simulink model "pendulum3"  (R2020b)
settings: Solver=VariableStepAuto  StartTime=0.0  StopTime=20  RelTol=1e-3
settings Model: Creator=Admin  LastModifiedBy=Admin

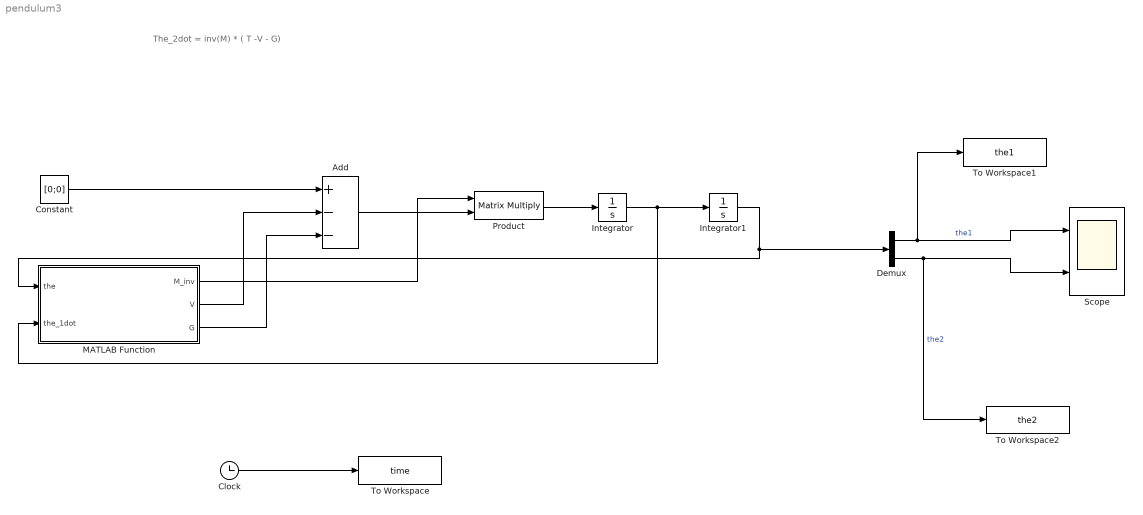
== system pendulum3 ==
  note: The_2dot = inv(M) * ( T -V - G)
  Add : Sum  Inputs=+--
  Clock : Clock
  Constant : Constant  Value=[0;0]  VectorParams1D=off
  Demux : Demux  Outputs=2
  Integrator : Integrator  InitialCondition=[0;0]
  Integrator1 : Integrator  InitialCondition=[pi/3;-pi/4]
  MATLAB Function : MATLAB Function  TreatAsAtomicUnit=on
  Product : Product  Multiplication=Matrix(*)
  Scope : Scope  NumInputPorts=2
  To Workspace : ToWorkspace  VariableName=time  SampleTime=-1
      settings: Save2DSignal=2-D array (concatenate along first dimension)
  To Workspace1 : ToWorkspace  VariableName=the1  SampleTime=-1
      settings: Save2DSignal=2-D array (concatenate along first dimension)
  To Workspace2 : ToWorkspace  VariableName=the2  SampleTime=-1
      settings: Save2DSignal=2-D array (concatenate along first dimension)
  wires:
  Constant/1 -> Add/1
  MATLAB Function/2(V) -> Add/2
  MATLAB Function/3(G) -> Add/3
  Add/1 -> Product/2
  MATLAB Function/1(M_inv) -> Product/1
  Product/1 -> Integrator/1
  Integrator/1 -> MATLAB Function/2(the_1dot), Integrator1/1
  Integrator1/1 -> Demux/1, MATLAB Function/1(the)
  Demux/1 -> To Workspace1/1, Scope/1  "the1"
  Demux/2 -> To Workspace2/1, Scope/2  "the2"
  Clock/1 -> To Workspace/1

== matlab function pendulum3/MATLAB Function ==
  data: the input; M_inv output; the_1dot input; V output; G output
function [M_inv, V, G]= fcn(the, the_1dot)

% robot parameters
m1 = 1;
m2 = 1;
l1 = 1;
l2 = 1;
g = 9.81;

c1 = cos(the(1));
c2 = cos(the(2));
s1 = sin(the(1));
s2 = sin(the(2));

M = [ l1^2*(m1+m2),  0;...
      0           ,    l2^2 * m2 ];
 
M_inv = inv(M);

V = the_1dot;

G = [0;...
   -m2*g*l2*c2];
